simulink model "mosfetbuckboost_avg"  (R2014a)
settings: Solver=ode23tb  StartTime=0.0  StopTime=10  FixedStep=1e-08  RelTol=1e-4
undefined symbols (not defined in the file or in its folder): Ts
libraries: powerlib x21, slctrlblks x2
settings Model: Creator=cosorio  LastModifiedBy=cosorio
settings DataIOCC: LimitDataPoints=off  SaveOutput=off  DSMLogging=off  SaveTime=off
settings OptimizationCC: ExpressionDepthLimit=2147483647
settings DebuggingCC: UnderspecifiedInitializationDetection=Classic  SolverPrmCheckMsg=none  FcnCallInpInsideContextMsg=UseLocalSettings  StateNameClashWarn=warning
settings GRTTargetCC: CombineOutputUpdateFcns=off  GRTInterface=on

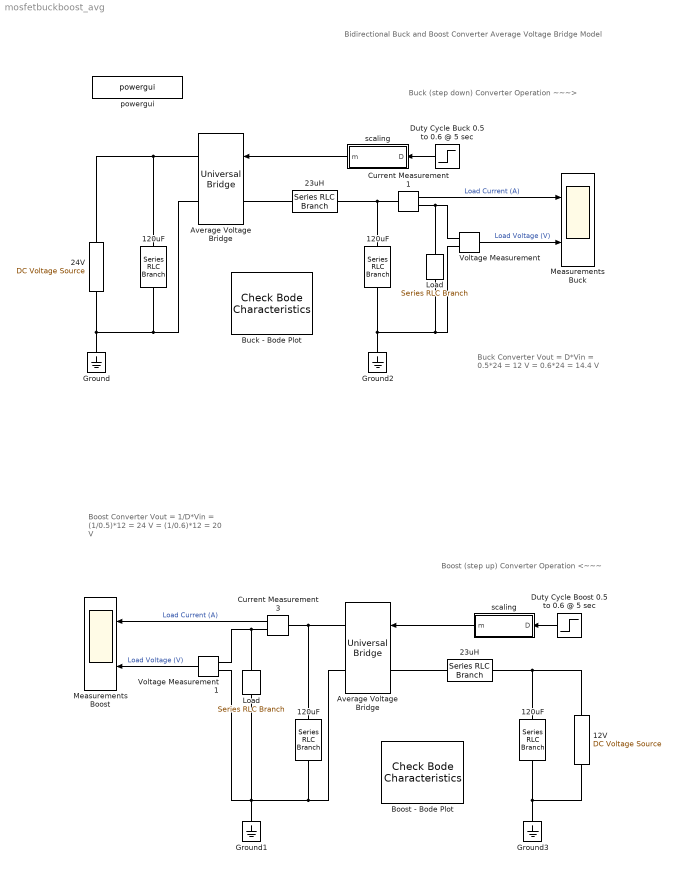
== system mosfetbuckboost_avg ==
  note: Bidirectional Buck and Boost Converter
      | Average Voltage Bridge Model
  note: Buck (step down) Converter Operation
      | ~~~>
  note: Boost (step up) Converter Operation
      | <~~~
  note: Boost Converter
      | Vout = 1/D*Vin
      | = (1/0.5)*12
      | = 24 V
      |
      | = (1/0.6)*12
      | = 20 V
  note: Buck Converter
      | Vout = D*Vin
      | = 0.5*24
      | = 12 V
      |
      | = 0.6*24
      | = 14.4 V
  "   120uF" : powerlib/Elements/Series RLC Branch  LConnTagsString=__new0  RConnTagsString=__new0  BranchType=RC  Resistance=0.005  Inductance=30e-6  SetiL0=off  InitialCurrent=0  Capacitance=120e-6  Setx0=on  InitialVoltage=12  Measurements=None
  "  120uF" : powerlib/Elements/Series RLC Branch  LConnTagsString=__new0  RConnTagsString=__new0  BranchType=RC  Resistance=0.005  Inductance=30e-6  SetiL0=off  InitialCurrent=0  Capacitance=120e-6  Setx0=on  InitialVoltage=24  Measurements=None
  " 120uF" : powerlib/Elements/Series RLC Branch  LConnTagsString=__new0  RConnTagsString=__new0  BranchType=RC  Resistance=0.005  Inductance=30e-6  SetiL0=off  InitialCurrent=0  Capacitance=120e-6  Setx0=on  InitialVoltage=24  Measurements=None
  " 23uH" : powerlib/Elements/Series RLC Branch  LConnTagsString=__new0  RConnTagsString=__new0  BranchType=RL  Resistance=0.001  Inductance=23e-6  SetiL0=on  InitialCurrent=48  Capacitance=1e-6  Setx0=off  InitialVoltage=0  Measurements=None
  120uF : powerlib/Elements/Series RLC Branch  LConnTagsString=__new0  RConnTagsString=__new0  BranchType=RC  Resistance=0.005  Inductance=30e-6  SetiL0=off  InitialCurrent=0  Capacitance=120e-6  Setx0=on  InitialVoltage=12  Measurements=None
  12V : powerlib/Electrical Sources/DC Voltage Source  Amplitude=12  Measurements=None
  23uH : powerlib/Elements/Series RLC Branch  LConnTagsString=__new0  RConnTagsString=__new0  BranchType=RL  Resistance=0.001  Inductance=23e-6  SetiL0=on  InitialCurrent=10  Capacitance=1e-6  Setx0=off  InitialVoltage=0  Measurements=None
  24V : powerlib/Electrical Sources/DC Voltage Source  Amplitude=24  Measurements=None
  Average Voltage Bridge : powerlib/Power Electronics/Universal Bridge  Arms=1  SnubberResistance=1e5  SnubberCapacitance=inf  Device=Average-model based VSC  Ron=1e-3  Lon=0  ForwardVoltages="[  0  0  ]"  ForwardVoltage=0  GTOparameters=[ 10e-6 , 20e-6 ]  IGBTparameters=[ 1e-6 , 2e-6 ]  Measurements=None  Measurements_2=None  converterType=Rectifier
  Average Voltage Bridge : powerlib/Power Electronics/Universal Bridge  Arms=1  SnubberResistance=1e5  SnubberCapacitance=inf  Device=Average-model based VSC  Ron=1e-3  Lon=0  ForwardVoltages="[  0  0  ]"  ForwardVoltage=0  GTOparameters=[ 10e-6 , 20e-6 ]  IGBTparameters=[ 1e-6 , 2e-6 ]  Measurements=None  Measurements_2=None  converterType=Rectifier
  Boost - Bode Plot : slctrlblks/Model Verification/Check Bode  Characteristics  InstantiateOnLoad=on  SaveOperatingPoints=off  LinearizationIOs={'/Duty Cycle Boost 0.5 to 0.6 @ 5 sec', 1, 'in', 'off', '';'/Voltage Measurement1', 1, 'out', 'off', ''}  LinearizeAt=SnapshotTimes  SnapshotTimes=[2,8]  TriggerType=rising  SampleTime=auto  RateConversionMethod=zoh  PreWarpFreq=10  UseExactDelayModel=off  UseFullBlockNameLabels=off  UseBusSignalLabels=off  enabled=on  stopWhenAssertionFail=off  export=off  ViewDlgPos=[528 32 505 532]  OpenViewOnLoad=off  LaunchViewOnOpen=on  FrequencyUnits=rad/s  MagnitudeUnits=dB  PhaseUnits=deg  TimeUnits=seconds  EnableUpperBound=off  UpperBoundFrequencies=[]  UpperBoundMagnitudes=[]  EnableLowerBound=off  LowerBoundFrequencies=[]  LowerBoundMagnitudes=[]
      settings: SaveToWorkspace=on  SaveName=sys_boost
  Buck - Bode Plot : slctrlblks/Model Verification/Check Bode  Characteristics  InstantiateOnLoad=on  SaveOperatingPoints=off  LinearizationIOs={'/Duty Cycle Buck 0.5 to 0.6 @ 5 sec', 1, 'in', 'off', '';'/Voltage Measurement', 1, 'out', 'off', ''}  LinearizeAt=SnapshotTimes  SnapshotTimes=[8]  TriggerType=rising  SampleTime=auto  RateConversionMethod=zoh  PreWarpFreq=10  UseExactDelayModel=off  UseFullBlockNameLabels=off  UseBusSignalLabels=off  enabled=on  stopWhenAssertionFail=off  export=off  ViewDlgPos=[7 30 504 534]  OpenViewOnLoad=off  LaunchViewOnOpen=on  FrequencyUnits=rad/s  MagnitudeUnits=dB  PhaseUnits=deg  TimeUnits=seconds  EnableUpperBound=off  UpperBoundFrequencies=[]  UpperBoundMagnitudes=[]  EnableLowerBound=off  LowerBoundFrequencies=[]  LowerBoundMagnitudes=[]
      settings: SaveToWorkspace=on  SaveName=sys_buck
  Current Measurement1 : powerlib/Measurements/Current Measurement  PhasorSimulation=off  OutputType=Complex  PSBequivalent=0
  Current Measurement3 : powerlib/Measurements/Current Measurement  PhasorSimulation=off  OutputType=Complex  PSBequivalent=0
  Duty Cycle Boost 0.5 to 0.6 @ 5 sec : Step  Time=5  Before=0.5  After=0.6  SampleTime=0
  Duty Cycle Buck 0.5 to 0.6 @ 5 sec : Step  Time=5  Before=0.5  After=0.6  SampleTime=0
  Ground{,1..3} (4 alike) : powerlib/Elements/Ground  LConnTagsString=a
  Load : powerlib/Elements/Series RLC Branch  LConnTagsString=__new0  RConnTagsString=__new0  BranchType=R  Resistance=1  Inductance=30e-6  SetiL0=off  InitialCurrent=0  Capacitance=100e-6  Setx0=off  InitialVoltage=0  Measurements=None
  "Load " : powerlib/Elements/Series RLC Branch  LConnTagsString=__new0  RConnTagsString=__new0  BranchType=R  Resistance=1  Inductance=30e-6  SetiL0=off  InitialCurrent=0  Capacitance=100e-6  Setx0=off  InitialVoltage=0  Measurements=None
  Measurements Boost : Scope  NumInputPorts=2
      settings: YMin=0~0  YMax=30~30
  Measurements Buck : Scope  NumInputPorts=2
      settings: YMin=0~0  YMax=20~20
  Voltage Measurement : powerlib/Measurements/Voltage Measurement  PhasorSimulation=off  OutputType=Complex  PSBequivalent=0
  Voltage Measurement1 : powerlib/Measurements/Voltage Measurement  PhasorSimulation=off  OutputType=Complex  PSBequivalent=0
  powergui : powerlib/powergui  Priority=1  SimulationMode=Continuous  SolverType=Tustin  SampleTime=Ts  frequency=60  SPID=off  DisableSnubberDevices=on  DisableRonSwitches=on  DisableVfSwitches=off  SwTol=0  Interpol=off  DisplayEquations=off  Ts=0  methode=off  frequencyindice=0  Pbase=100e6  ErrMax=1e-4  Iterations=50  UnitsV=kV  UnitsW=MW  FunctionMessages=off  echomessages=off  HookPort=off  EnableUseOfTLC=off  x0status=blocks  RestoreLinks=warning  ResistiveCurrentMeasurement=off  Frange=[0:2:500]  Ylog=off  Xlog=on  ShowGrid=off  save=off  variable=ZData  structure=0  ZoomFFT=on  StartTime=0.0  cycles=1  DisplayStyle=1  fundamental=60  FreqAxis=off  MaxFrequency=1000  frequencyindicesteady=1  RmsSteady=1  display=off
  scaling : Subsystem
  "scaling " : Subsystem
  wires:
  Voltage Measurement1/1 -> Measurements Boost/2  "Load Voltage (V)"
  Current Measurement3/1 -> Measurements Boost/1  "Load Current (A)"
  Current Measurement1/1 -> Measurements Buck/1  "Load Current (A)"
  Voltage Measurement/1 -> Measurements Buck/2  "Load Voltage (V)"
  Duty Cycle Buck 0.5 to 0.6 @ 5 sec/1 -> scaling/1(D)
  scaling/1(m) -> Average Voltage Bridge/1
  Duty Cycle Boost 0.5 to 0.6 @ 5 sec/1 -> "scaling "/1(D)
  "scaling "/1(m) -> Average Voltage Bridge/1
  connections:
  Average Voltage Bridge/RConn2 -- " 120uF"/RConn1 -- Ground/LConn1 -- 24V/LConn1
  23uH/LConn1 -- 120uF/LConn1 -- Current Measurement1/LConn1
  " 120uF"/LConn1 -- 24V/RConn1 -- Average Voltage Bridge/RConn1
  12V/LConn1 -- "   120uF"/RConn1 -- Ground3/LConn1
  Voltage Measurement1/LConn1 -- "Load "/RConn1 -- Current Measurement3/RConn1
  12V/RConn1 -- "   120uF"/LConn1 -- " 23uH"/LConn1
  Current Measurement3/LConn1 -- "  120uF"/LConn1 -- Average Voltage Bridge/RConn1
  Load/RConn1 -- Current Measurement1/RConn1 -- Voltage Measurement/LConn1
  Average Voltage Bridge/LConn1 -- 23uH/RConn1
  120uF/RConn1 -- Load/LConn1 -- Voltage Measurement/LConn2 -- Ground2/LConn1
  Average Voltage Bridge/LConn1 -- " 23uH"/RConn1
  Average Voltage Bridge/RConn2 -- "  120uF"/RConn1 -- Ground1/LConn1 -- "Load "/LConn1 -- Voltage Measurement1/LConn2

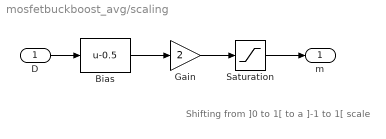
== system mosfetbuckboost_avg/scaling ==
  note: Shifting from ]0 to 1[ to a ]-1 to 1[ scale
  D : Inport
  Bias : Bias  Bias=-0.5
  Gain : Gain  Gain=2
  Saturation : Saturate  UpperLimit=1  LowerLimit=-1
  m : Outport
  wires:
  Bias/1 -> Gain/1
  D/1 -> Bias/1
  Gain/1 -> Saturation/1
  Saturation/1 -> m/1

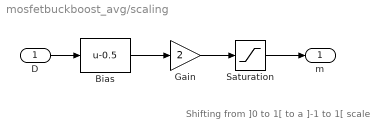
== system mosfetbuckboost_avg/scaling  ==
  note: Shifting from ]0 to 1[ to a ]-1 to 1[ scale
  D : Inport
  Bias : Bias  Bias=-0.5
  Gain : Gain  Gain=2
  Saturation : Saturate  UpperLimit=1  LowerLimit=-1
  m : Outport
  wires:
  Bias/1 -> Gain/1
  D/1 -> Bias/1
  Gain/1 -> Saturation/1
  Saturation/1 -> m/1
